simulink library "lib_abs_nodiv"  (Simulink 7.7)
settings: Solver=ode45  SolverMode=SingleTasking  StartTime=0.0  StopTime=10.0  RelTol=1e-3
undefined symbols (not defined in the file): R, slip_abs_on
settings Model: Creator=yt59680  LastModifiedBy=lfeng

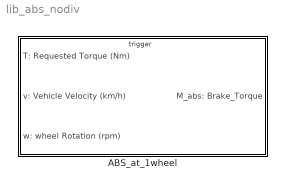
== system lib_abs_nodiv ==
  ABS_at_1wheel : Subsystem  TreatAsAtomicUnit=on

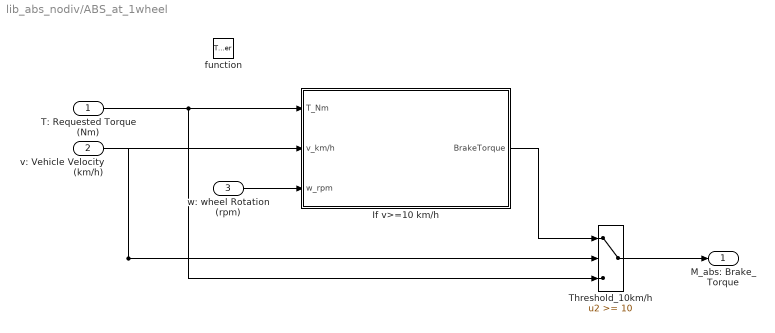
== system lib_abs_nodiv/ABS_at_1wheel ==
  T: Requested Torque (Nm) : Inport
  v: Vehicle Velocity (km/h) : Inport  Port=2
  w: wheel Rotation (rpm) : Inport  Port=3
  function : TriggerPort  TriggerType=function-call
  If v>=10 km/h : Subsystem  TreatAsAtomicUnit=on
  Threshold_10km/h : Switch  Threshold=10
  M_abs: Brake_Torque : Outport
  wires:
  w: wheel Rotation (rpm)/1 -> If v>=10 km/h/3(w_rpm)
  Threshold_10km/h/1 -> M_abs: Brake_Torque/1
  If v>=10 km/h/1(BrakeTorque) -> Threshold_10km/h/1
  T: Requested Torque (Nm)/1 -> If v>=10 km/h/1(T_Nm), Threshold_10km/h/3
  v: Vehicle Velocity (km/h)/1 -> If v>=10 km/h/2(v_km/h), Threshold_10km/h/2

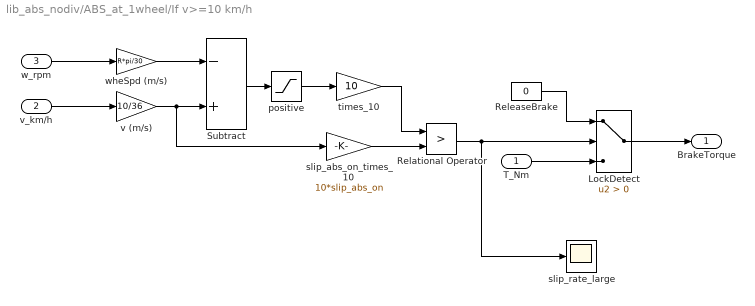
== system lib_abs_nodiv/ABS_at_1wheel/If v>=10 km/h ==
  T_Nm : Inport
  v_km/h : Inport  Port=2
  w_rpm : Inport  Port=3
  LockDetect : Switch  Criteria=u2 > Threshold
  Relational Operator : RelationalOperator  Operator=>  OutDataTypeStr=boolean
  ReleaseBrake : Constant  Value=0  OutDataTypeStr=uint8
  Subtract : Sum  Inputs=-+
  positive : Saturate  UpperLimit=inf  LowerLimit=0
  slip_abs_on_times_10 : Gain  Gain=10*slip_abs_on
  slip_rate_large : Scope
      settings: SaveName=ScopeData7
  times_10 : Gain  Gain=10
  v (m/s) : Gain  Gain=10/36  OutMin=0  OutMax=100
  wheSpd (m/s) : Gain  Gain=R*pi/30  OutMin=0  OutMax=100
  BrakeTorque : Outport
  wires:
  positive/1 -> times_10/1
  slip_abs_on_times_10/1 -> Relational Operator/2
  w_rpm/1 -> wheSpd (m/s)/1
  v_km/h/1 -> v (m/s)/1
  Subtract/1 -> positive/1
  times_10/1 -> Relational Operator/1
  Relational Operator/1 -> slip_rate_large/1, LockDetect/2
  LockDetect/1 -> BrakeTorque/1
  ReleaseBrake/1 -> LockDetect/1
  T_Nm/1 -> LockDetect/3
  wheSpd (m/s)/1 -> Subtract/1
  v (m/s)/1 -> slip_abs_on_times_10/1, Subtract/2
